simulink model "mdl_4reac"  (R2020b)
settings: Solver=FixedStepAuto  StartTime=0.0  StopTime=stoptime  FixedStep=0.001  MaxStep=1  RelTol=1e-3  AbsTol=1e-6
undefined symbols (not defined in the file or in its folder): p, ref_select, strategy_select
(part 1 of 2)
settings Model: PauseTimes=3  PacingRate=0.100000  Creator=nobel  LastModifiedBy=natha

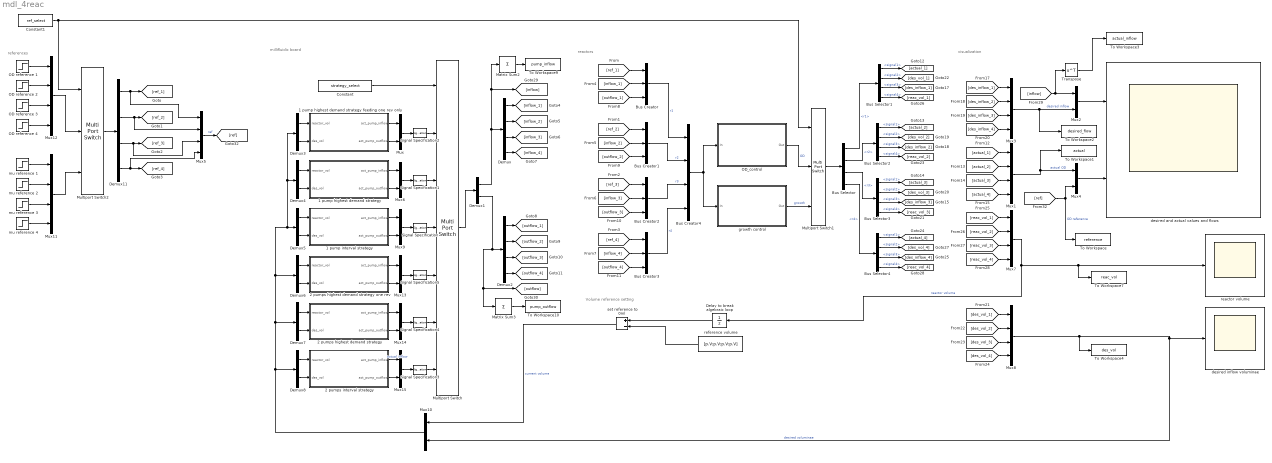
== system mdl_4reac ==
  note: millifluidic board
  note: references
  note: Volume reference setting
  note: visualization
  note: reactors
  " 1 pump highest demand strategy" : Stateflow chart  TreatAsAtomicUnit=on  mask{p=p}
      mask prompts: p "Reactor Parameter Struct"
  " 1 pump highest demand strategy feeding one rev only" : Stateflow chart  TreatAsAtomicUnit=on  mask{p=p}
      mask prompts: p "Reactor Parameter Struct"
  1 pump interval strategy : Stateflow chart  TreatAsAtomicUnit=on  mask{p=p}
      mask prompts: p "Reactor Parameter Struct"
  2 pumps highest demand strategy : Stateflow chart  TreatAsAtomicUnit=on  mask{p=p}
      mask prompts: p "Reactor Parameter Struct"
  2 pumps highest demand strategy one rev : Stateflow chart  TreatAsAtomicUnit=on  mask{p=p}
      mask prompts: p "Reactor Parameter Struct"
  2 pumps interval strategy : Stateflow chart  TreatAsAtomicUnit=on  mask{p=p}
      mask prompts: p "Reactor Parameter Struct"
  Bus Creator{,1..3} (4 alike) : BusCreator  Inputs=3
  Bus Creator4 : BusCreator  Inputs=4
  Bus Selector : BusSelector  OutputSignals=r1,r2,r3,r4
  Bus Selector{1..4} (4 alike) : BusSelector  OutputSignals=signal1,signal2,signal3,signal4
  Constant : Constant  Value=strategy_select
  Constant1 : Constant  Value=ref_select
  Delay to break algebraic loop : UnitDelay  InitialCondition=[15; 15; 15; 15]  SampleTime=-1  HasFrameUpgradeWarning=on
  Demux : Demux
  Demux{1,3..8} (7 alike) : Demux  Outputs=2
  Demux11 : Demux
  Demux2 : Demux
  Matrix Sum2 : Sum  Inputs=+
  Matrix Sum3 : Sum  Inputs=+
  Multiport Switch : MultiPortSwitch  Inputs=6
  Multiport Switch1 : MultiPortSwitch  Inputs=2
  Multiport Switch2 : MultiPortSwitch  Inputs=2
  Mux{,2,4,6,9..10,13..15} (9 alike) : Mux  Inputs=2
  Mux{1,3,5,7..8,11..12} (7 alike) : Mux
  OD reference 1 : Step  Time=p.r1_OD.step_time  Before=p.r1_OD.init_val  After=p.r1_OD.final_val  SampleTime=0  mask{p=p}
      mask prompts: p "Reactor Parameter Struct"
  OD reference 2 : Step  Time=p.r2_OD.step_time  Before=p.r2_OD.init_val  After=p.r2_OD.final_val  SampleTime=0  mask{p=p}
      mask prompts: p "Reactor Parameter Struct"
  OD reference 3 : Step  Time=p.r3_OD.step_time  Before=p.r3_OD.init_val  After=p.r3_OD.final_val  SampleTime=0  mask{p=p}
      mask prompts: p "Reactor Parameter Struct"
  OD reference 4 : Step  Time=p.r4_OD.step_time  Before=p.r4_OD.init_val  After=p.r4_OD.final_val  SampleTime=0  mask{p=p}
      mask prompts: p "Reactor Parameter Struct"
  OD_control : Subsystem
  Signal Specification{,1..5} (6 alike) : SignalSpecification  Dimensions=[8 1]
  To Workspace : ToWorkspace  VariableName=reference  SampleTime=-1
  To Workspace1 : ToWorkspace  VariableName=actual  SampleTime=-1
  To Workspace10 : ToWorkspace  VariableName=pump_outflow  SampleTime=-1
      settings: Save2DSignal=2-D array (concatenate along first dimension)
  To Workspace2 : ToWorkspace  VariableName=desired_flow  SampleTime=-1
  To Workspace3 : ToWorkspace  VariableName=actual_inflow  SampleTime=-1
      settings: Save2DSignal=2-D array (concatenate along first dimension)
  To Workspace4 : ToWorkspace  VariableName=des_vol  SampleTime=-1
  To Workspace7 : ToWorkspace  VariableName=reac_vol  SampleTime=-1
  To Workspace9 : ToWorkspace  VariableName=pump_inflow  SampleTime=-1
      settings: Save2DSignal=2-D array (concatenate along first dimension)
  Transpose : Math  Operator=transpose  SaturateOnIntegerOverflow=on
  desired and actual values and flows : Scope  NumInputPorts=2
  desired inflow voluminae : Scope
  growth control : Subsystem
  mu reference 1 : Step  Time=p.r1_growth.step_time  Before=p.r1_growth.init_val  After=p.r1_growth.final_val  SampleTime=0  mask{p=p}
      mask prompts: p "Reactor Parameter Struct"
  mu reference 2 : Step  Time=p.r2_growth.step_time  Before=p.r2_growth.init_val  After=p.r2_growth.final_val  SampleTime=0  mask{p=p}
      mask prompts: p "Reactor Parameter Struct"
  mu reference 3 : Step  Time=p.r3_growth.step_time  Before=p.r3_growth.init_val  After=p.r3_growth.final_val  SampleTime=0  mask{p=p}
      mask prompts: p "Reactor Parameter Struct"
  mu reference 4 : Step  Time=p.r4_growth.step_time  Before=p.r4_growth.init_val  After=p.r4_growth.final_val  SampleTime=0  mask{p=p}
      mask prompts: p "Reactor Parameter Struct"
  reactor volume : Scope
  reference volume : Constant  Value=[p.V;p.V;p.V;p.V]  mask{p=p}
      mask prompts: p "Reactor Parameter Struct"
  set reference to 0ml : Sum  Inputs=+-
  wires:
  Mux5/1 -> [ref]  "ref"
  Demux11/1 -> Mux5/1, [ref_1]
  Demux11/2 -> Mux5/2, [ref_2]
  Demux11/3 -> Mux5/3, [ref_3]
  Demux11/4 -> Mux5/4, [ref_4]
  Demux/1 -> [inflow_1]
  Demux/2 -> [inflow_2]
  Demux/3 -> [inflow_3]
  Demux/4 -> [inflow_4]
  Demux2/4 -> [outflow_4]
  Demux2/3 -> [outflow_3]
  Demux2/2 -> [outflow_2]
  Demux2/1 -> [outflow_1]
  Demux1/2 -> Matrix Sum3/1, [outflow], Demux2/1
  Matrix Sum2/1 -> To Workspace9/1
  Demux1/1 -> Matrix Sum2/1, [inflow], Demux/1
  Matrix Sum3/1 -> To Workspace10/1
  [des_vol_3] -> Mux8/3
  [ref] -> To Workspace/1, Mux4/2  "OD reference"
  Mux3/1 -> To Workspace2/1, Mux2/2  "desired inflow"
  Delay to break algebraic loop/1 -> set reference to 0ml/1
  Mux8/1 -> To Workspace4/1, Mux10/2, desired inflow voluminae/1  "desired voluminae"
  [des_vol_2] -> Mux8/2
  [reac_vol_1] -> Mux7/1
  [reac_vol_3] -> Mux7/3
  [actual_1] -> Mux1/1
  [actual_4] -> Mux1/4
  Mux4/1 -> desired and actual values and flows/2
  [des_inflow_3] -> Mux3/3
  [des_inflow_2] -> Mux3/2
  reference volume/1 -> set reference to 0ml/2
  Mux1/1 -> To Workspace1/1, Mux4/1  "actual OD"
  [reac_vol_2] -> Mux7/2
  [des_vol_4] -> Mux8/4
  [actual_2] -> Mux1/2
  [inflow] -> Transpose/1, Mux2/1
  [actual_3] -> Mux1/3
  [des_inflow_1] -> Mux3/1
  [reac_vol_4] -> Mux7/4
  set reference to 0ml/1 -> Mux10/1  "current volume"
  [des_vol_1] -> Mux8/1
  Mux2/1 -> desired and actual values and flows/1
  Mux7/1 -> Delay to break algebraic loop/1, To Workspace7/1, reactor volume/1  "reactor volume"
  [des_inflow_4] -> Mux3/4
  Transpose/1 -> To Workspace3/1
  Mux6/1 -> Signal Specification1/1
  Mux/1 -> Signal Specification2/1
  Demux5/1 -> 1 pump interval strategy/1(reactor_vol)
  Demux4/1 -> " 1 pump highest demand strategy"/1(reactor_vol)
  " 1 pump highest demand strategy"/2(act_pump_outflow) -> Mux6/2
  Demux3/2 -> " 1 pump highest demand strategy feeding one rev only"/2(des_vol)
  1 pump interval strategy/1(act_pump_inflow) -> Mux9/1
  " 1 pump highest demand strategy feeding one rev only"/2(act_pump_outflow) -> Mux/2
  " 1 pump highest demand strategy feeding one rev only"/1(act_pump_inflow) -> Mux/1
  1 pump interval strategy/2(act_pump_outflow) -> Mux9/2
  Demux4/2 -> " 1 pump highest demand strategy"/2(des_vol)
  Demux3/1 -> " 1 pump highest demand strategy feeding one rev only"/1(reactor_vol)
  " 1 pump highest demand strategy"/1(act_pump_inflow) -> Mux6/1
  Demux5/2 -> 1 pump interval strategy/2(des_vol)
  Mux9/1 -> Signal Specification/1
  Constant/1 -> Multiport Switch/1
  Bus Selector3/4 -> [reac_vol_3]  "<signal4>"
  Bus Selector4/2 -> [des_vol_4]  "<signal2>"
  Bus Selector3/2 -> [des_vol_3]  "<signal2>"
  Bus Selector1/1 -> [actual_1]  "<signal1>"
  Bus Selector2/3 -> [des_inflow_2]  "<signal3>"
  Bus Selector1/2 -> [des_vol_1]  "<signal2>"
  Bus Selector1/4 -> [reac_vol_1]  "<signal4>"
  Bus Selector1/3 -> [des_inflow_1]  "<signal3>"
  Bus Selector3/3 -> [des_inflow_3]  "<signal3>"
  Bus Selector4/4 -> [reac_vol_4]  "<signal4>"
  Bus Selector2/4 -> [reac_vol_2]  "<signal4>"
  Bus Selector4/3 -> [des_inflow_4]  "<signal3>"
  Bus Selector4/1 -> [actual_4]  "<signal1>"
  Bus Selector3/1 -> [actual_3]  "<signal1>"
  Bus Selector2/1 -> [actual_2]  "<signal1>"
  Bus Selector2/2 -> [des_vol_2]  "<signal2>"
  Bus Selector/2 -> Bus Selector2/1  "<r2>"
  Bus Selector/4 -> Bus Selector4/1  "<r4>"
  [inflow_4] -> Bus Creator3/2
  [inflow_2] -> Bus Creator1/2
  [inflow_1] -> Bus Creator/2
  [inflow_3] -> Bus Creator2/2
  [outflow_3] -> Bus Creator2/3
  [ref_2] -> Bus Creator1/1
  [outflow_1] -> Bus Creator/3
  [ref_1] -> Bus Creator/1
  [outflow_4] -> Bus Creator3/3
  [ref_4] -> Bus Creator3/1
  [ref_3] -> Bus Creator2/1
  [outflow_2] -> Bus Creator1/3
  OD reference 1/1 -> Mux12/1
  OD reference 2/1 -> Mux12/2
  OD reference 3/1 -> Mux12/3
  OD reference 4/1 -> Mux12/4
  mu reference 4/1 -> Mux11/4
  mu reference 3/1 -> Mux11/3
  mu reference 2/1 -> Mux11/2
  mu reference 1/1 -> Mux11/1
  Multiport Switch2/1 -> Demux11/1
  Mux12/1 -> Multiport Switch2/2
  Mux11/1 -> Multiport Switch2/3
  Constant1/1 -> Multiport Switch2/1, Multiport Switch1/1
  Bus Creator/1 -> Bus Creator4/1  "r1"
  Bus Creator1/1 -> Bus Creator4/2  "r2"
  Bus Creator2/1 -> Bus Creator4/3  "r3"
  Bus Creator3/1 -> Bus Creator4/4  "r4"
  Bus Creator4/1 -> growth control/1(In), OD_control/1(In)
  Multiport Switch/1 -> Demux1/1
  Bus Selector/1 -> Bus Selector1/1  "<r1>"
  Bus Selector/3 -> Bus Selector3/1  "<r3>"
  growth control/1(Out) -> Multiport Switch1/3  "growth"
  OD_control/1(Out) -> Multiport Switch1/2  "OD"
  Multiport Switch1/1 -> Bus Selector/1
  Signal Specification/1 -> Multiport Switch/4
  Signal Specification1/1 -> Multiport Switch/3
  Signal Specification2/1 -> Multiport Switch/2
  Demux7/2 -> 2 pumps highest demand strategy/2(des_vol)
  Demux8/1 -> 2 pumps interval strategy/1(reactor_vol)
  Demux6/2 -> 2 pumps highest demand strategy one rev/2(des_vol)
  Mux14/1 -> Signal Specification4/1
  2 pumps highest demand strategy/1(act_pump_inflow) -> Mux14/1
  2 pumps interval strategy/2(act_pump_outflow) -> Mux15/2
  Mux15/1 -> Signal Specification3/1
  Demux7/1 -> 2 pumps highest demand strategy/1(reactor_vol)
  2 pumps highest demand strategy one rev/1(act_pump_inflow) -> Mux13/1
  Mux10/1 -> Demux8/1, Demux7/1, Demux6/1, Demux5/1, Demux4/1, Demux3/1
  2 pumps highest demand strategy/2(act_pump_outflow) -> Mux14/2
  Demux6/1 -> 2 pumps highest demand strategy one rev/1(reactor_vol)
  Demux8/2 -> 2 pumps interval strategy/2(des_vol)
  2 pumps highest demand strategy one rev/2(act_pump_outflow) -> Mux13/2
  2 pumps interval strategy/1(act_pump_inflow) -> Mux15/1  "actual inflow"
  Mux13/1 -> Signal Specification5/1
  Signal Specification3/1 -> Multiport Switch/7
  Signal Specification5/1 -> Multiport Switch/5
  Signal Specification4/1 -> Multiport Switch/6

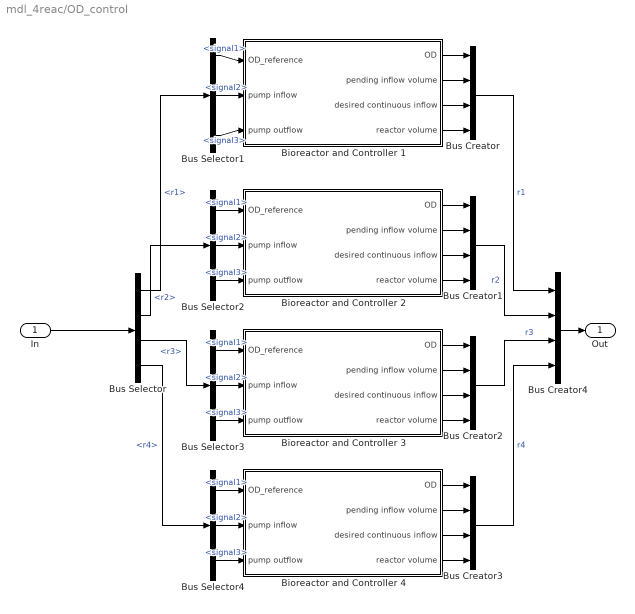
== system mdl_4reac/OD_control ==
  In : Inport
  Bioreactor and Controller 1 : Subsystem  mask{p=p}
      mask prompts: p "Reactor Parameter Struct"
  Bioreactor and Controller 2 : Subsystem  mask{p=p}
      mask prompts: p "Reactor Parameter Struct"
  Bioreactor and Controller 3 : Subsystem  mask{p=p}
      mask prompts: p "Reactor Parameter Struct"
  Bioreactor and Controller 4 : Subsystem  mask{p=p}
      mask prompts: p "Reactor Parameter Struct"
  Bus Creator{,1..4} (5 alike) : BusCreator  Inputs=4
  Bus Selector : BusSelector  OutputSignals=r1,r2,r3,r4
  Bus Selector{1..4} (4 alike) : BusSelector  OutputSignals=signal1,signal2,signal3
  Out : Outport
  wires:
  Bus Selector4/1 -> Bioreactor and Controller 4/1(OD_reference)  "<signal1>"
  Bus Selector/1 -> Bus Selector1/1  "<r1>"
  Bus Selector2/2 -> Bioreactor and Controller 2/2(pump inflow)  "<signal2>"
  Bus Creator3/1 -> Bus Creator4/4  "r4"
  Bioreactor and Controller 4/2(pending inflow volume) -> Bus Creator3/2
  Bus Selector1/2 -> Bioreactor and Controller 1/2(pump inflow)  "<signal2>"
  Bus Selector3/2 -> Bioreactor and Controller 3/2(pump inflow)  "<signal2>"
  Bus Selector/2 -> Bus Selector2/1  "<r2>"
  Bus Selector1/3 -> Bioreactor and Controller 1/3(pump outflow)  "<signal3>"
  Bus Creator4/1 -> Out/1
  Bus Selector/4 -> Bus Selector4/1  "<r4>"
  Bioreactor and Controller 2/4(reactor volume) -> Bus Creator1/4
  Bioreactor and Controller 2/1(OD) -> Bus Creator1/1
  Bioreactor and Controller 4/4(reactor volume) -> Bus Creator3/4
  Bus Selector2/3 -> Bioreactor and Controller 2/3(pump outflow)  "<signal3>"
  Bus Selector3/3 -> Bioreactor and Controller 3/3(pump outflow)  "<signal3>"
  Bioreactor and Controller 3/3(desired continuous inflow) -> Bus Creator2/3
  Bioreactor and Controller 1/1(OD) -> Bus Creator/1
  Bus Selector1/1 -> Bioreactor and Controller 1/1(OD_reference)  "<signal1>"
  Bioreactor and Controller 4/3(desired continuous inflow) -> Bus Creator3/3
  Bioreactor and Controller 2/3(desired continuous inflow) -> Bus Creator1/3
  Bus Selector3/1 -> Bioreactor and Controller 3/1(OD_reference)  "<signal1>"
  Bioreactor and Controller 3/4(reactor volume) -> Bus Creator2/4
  Bioreactor and Controller 4/1(OD) -> Bus Creator3/1
  Bioreactor and Controller 1/4(reactor volume) -> Bus Creator/4
  Bioreactor and Controller 3/2(pending inflow volume) -> Bus Creator2/2
  Bioreactor and Controller 3/1(OD) -> Bus Creator2/1
  Bioreactor and Controller 1/2(pending inflow volume) -> Bus Creator/2
  Bus Creator2/1 -> Bus Creator4/3  "r3"
  Bus Creator/1 -> Bus Creator4/1  "r1"
  Bus Selector4/3 -> Bioreactor and Controller 4/3(pump outflow)  "<signal3>"
  Bus Selector4/2 -> Bioreactor and Controller 4/2(pump inflow)  "<signal2>"
  Bus Selector/3 -> Bus Selector3/1  "<r3>"
  Bioreactor and Controller 1/3(desired continuous inflow) -> Bus Creator/3
  Bioreactor and Controller 2/2(pending inflow volume) -> Bus Creator1/2
  Bus Creator1/1 -> Bus Creator4/2  "r2"
  In/1 -> Bus Selector/1
  Bus Selector2/1 -> Bioreactor and Controller 2/1(OD_reference)  "<signal1>"

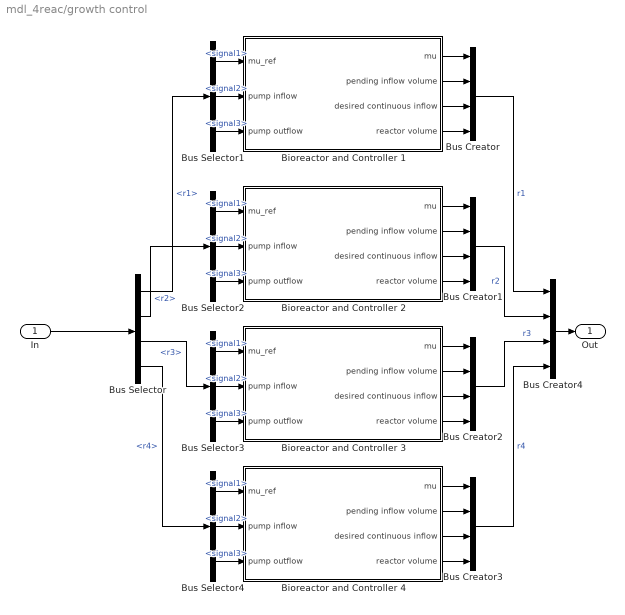
== system mdl_4reac/growth control ==
  In : Inport
  Bioreactor and Controller 1 : Subsystem  mask{p=p}
      mask prompts: p "Reactor Parameter Struct"
  Bioreactor and Controller 2 : Subsystem  mask{p=p}
      mask prompts: p "Reactor Parameter Struct"
  Bioreactor and Controller 3 : Subsystem  mask{p=p}
      mask prompts: p "Reactor Parameter Struct"
  Bioreactor and Controller 4 : Subsystem  mask{p=p}
      mask prompts: p "Reactor Parameter Struct"
  Bus Creator{,1..4} (5 alike) : BusCreator  Inputs=4
  Bus Selector : BusSelector  OutputSignals=r1,r2,r3,r4
  Bus Selector{1..4} (4 alike) : BusSelector  OutputSignals=signal1,signal2,signal3
  Out : Outport
  wires:
  Bus Creator2/1 -> Bus Creator4/3  "r3"
  Bus Creator/1 -> Bus Creator4/1  "r1"
  Bus Creator1/1 -> Bus Creator4/2  "r2"
  Bus Selector/3 -> Bus Selector3/1  "<r3>"
  In/1 -> Bus Selector/1
  Bus Selector2/3 -> Bioreactor and Controller 2/3(pump outflow)  "<signal3>"
  Bioreactor and Controller 3/2(pending inflow volume) -> Bus Creator2/2
  Bus Selector3/3 -> Bioreactor and Controller 3/3(pump outflow)  "<signal3>"
  Bioreactor and Controller 3/4(reactor volume) -> Bus Creator2/4
  Bioreactor and Controller 3/3(desired continuous inflow) -> Bus Creator2/3
  Bus Selector3/1 -> Bioreactor and Controller 3/1(mu_ref)  "<signal1>"
  Bus Selector3/2 -> Bioreactor and Controller 3/2(pump inflow)  "<signal2>"
  Bioreactor and Controller 2/2(pending inflow volume) -> Bus Creator1/2
  Bus Selector2/2 -> Bioreactor and Controller 2/2(pump inflow)  "<signal2>"
  Bus Selector2/1 -> Bioreactor and Controller 2/1(mu_ref)  "<signal1>"
  Bioreactor and Controller 2/3(desired continuous inflow) -> Bus Creator1/3
  Bioreactor and Controller 2/4(reactor volume) -> Bus Creator1/4
  Bioreactor and Controller 2/1(mu) -> Bus Creator1/1
  Bus Selector/4 -> Bus Selector4/1  "<r4>"
  Bioreactor and Controller 4/4(reactor volume) -> Bus Creator3/4
  Bioreactor and Controller 4/3(desired continuous inflow) -> Bus Creator3/3
  Bioreactor and Controller 4/2(pending inflow volume) -> Bus Creator3/2
  Bus Selector1/1 -> Bioreactor and Controller 1/1(mu_ref)  "<signal1>"
  Bus Selector4/1 -> Bioreactor and Controller 4/1(mu_ref)  "<signal1>"
  Bus Selector4/3 -> Bioreactor and Controller 4/3(pump outflow)  "<signal3>"
  Bus Selector4/2 -> Bioreactor and Controller 4/2(pump inflow)  "<signal2>"
  Bioreactor and Controller 4/1(mu) -> Bus Creator3/1
  Bioreactor and Controller 1/4(reactor volume) -> Bus Creator/4
  Bioreactor and Controller 1/3(desired continuous inflow) -> Bus Creator/3
  Bioreactor and Controller 1/1(mu) -> Bus Creator/1
  Bus Selector1/2 -> Bioreactor and Controller 1/2(pump inflow)  "<signal2>"
  Bus Selector/1 -> Bus Selector1/1  "<r1>"
  Bus Creator3/1 -> Bus Creator4/4  "r4"
  Bus Selector/2 -> Bus Selector2/1  "<r2>"
  Bus Selector1/3 -> Bioreactor and Controller 1/3(pump outflow)  "<signal3>"
  Bioreactor and Controller 1/2(pending inflow volume) -> Bus Creator/2
  Bioreactor and Controller 3/1(mu) -> Bus Creator2/1
  Bus Creator4/1 -> Out/1

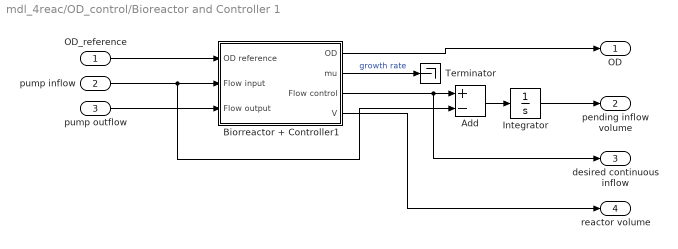
== system mdl_4reac/OD_control/Bioreactor and Controller 1 ==
  OD_reference : Inport
  pump inflow : Inport  Port=2
  pump outflow : Inport  Port=3
  Add : Sum  Inputs=+-
  Biorreactor + Controller1 : Subsystem
  Integrator : Integrator
  Terminator : Terminator
  OD : Outport
  pending inflow volume : Outport  Port=2
  desired continuous inflow : Outport  Port=3
  reactor volume : Outport  Port=4
  wires:
  OD_reference/1 -> Biorreactor + Controller1/1(OD reference)
  Biorreactor + Controller1/2(mu) -> Terminator/1  "growth rate"
  Biorreactor + Controller1/1(OD) -> OD/1
  Biorreactor + Controller1/3(Flow control) -> desired continuous inflow/1, Add/1
  pump inflow/1 -> Add/2, Biorreactor + Controller1/2(Flow input)
  Biorreactor + Controller1/4(V) -> reactor volume/1
  pump outflow/1 -> Biorreactor + Controller1/3(Flow output)
  Add/1 -> Integrator/1
  Integrator/1 -> pending inflow volume/1

== system mdl_4reac/OD_control/Bioreactor and Controller 2 ==
  OD_reference : Inport
  pump inflow : Inport  Port=2
  pump outflow : Inport  Port=3
  Add : Sum  Inputs=+-
  Biorreactor + Controller1 : Subsystem
  Integrator : Integrator
  Terminator : Terminator
  OD : Outport
  pending inflow volume : Outport  Port=2
  desired continuous inflow : Outport  Port=3
  reactor volume : Outport  Port=4
  wires:
  Integrator/1 -> pending inflow volume/1
  Add/1 -> Integrator/1
  pump outflow/1 -> Biorreactor + Controller1/3(Flow output)
  Biorreactor + Controller1/4(V) -> reactor volume/1
  pump inflow/1 -> Biorreactor + Controller1/2(Flow input), Add/2
  Biorreactor + Controller1/3(Flow control) -> Add/1, desired continuous inflow/1
  Biorreactor + Controller1/1(OD) -> OD/1
  Biorreactor + Controller1/2(mu) -> Terminator/1  "growth rate"
  OD_reference/1 -> Biorreactor + Controller1/1(OD reference)

== system mdl_4reac/OD_control/Bioreactor and Controller 3 ==
  OD_reference : Inport
  pump inflow : Inport  Port=2
  pump outflow : Inport  Port=3
  Add : Sum  Inputs=+-
  Biorreactor + Controller1 : Subsystem
  Integrator : Integrator
  Terminator : Terminator
  OD : Outport
  pending inflow volume : Outport  Port=2
  desired continuous inflow : Outport  Port=3
  reactor volume : Outport  Port=4
  wires:
  OD_reference/1 -> Biorreactor + Controller1/1(OD reference)
  Biorreactor + Controller1/2(mu) -> Terminator/1  "growth rate"
  Biorreactor + Controller1/1(OD) -> OD/1
  Biorreactor + Controller1/3(Flow control) -> desired continuous inflow/1, Add/1
  pump inflow/1 -> Add/2, Biorreactor + Controller1/2(Flow input)
  Biorreactor + Controller1/4(V) -> reactor volume/1
  pump outflow/1 -> Biorreactor + Controller1/3(Flow output)
  Add/1 -> Integrator/1
  Integrator/1 -> pending inflow volume/1

== system mdl_4reac/OD_control/Bioreactor and Controller 4 ==
  OD_reference : Inport
  pump inflow : Inport  Port=2
  pump outflow : Inport  Port=3
  Add : Sum  Inputs=+-
  Biorreactor + Controller1 : Subsystem
  Integrator : Integrator
  Terminator : Terminator
  OD : Outport
  pending inflow volume : Outport  Port=2
  desired continuous inflow : Outport  Port=3
  reactor volume : Outport  Port=4
  wires:
  Integrator/1 -> pending inflow volume/1
  Add/1 -> Integrator/1
  pump outflow/1 -> Biorreactor + Controller1/3(Flow output)
  Biorreactor + Controller1/4(V) -> reactor volume/1
  pump inflow/1 -> Biorreactor + Controller1/2(Flow input), Add/2
  Biorreactor + Controller1/3(Flow control) -> Add/1, desired continuous inflow/1
  Biorreactor + Controller1/1(OD) -> OD/1
  Biorreactor + Controller1/2(mu) -> Terminator/1  "growth rate"
  OD_reference/1 -> Biorreactor + Controller1/1(OD reference)

== system mdl_4reac/growth control/Bioreactor and Controller 1 ==
  mu_ref : Inport
  pump inflow : Inport  Port=2
  pump outflow : Inport  Port=3
  Add : Sum  Inputs=+-
  Biorreactor + Controller 1 : Subsystem
  Integrator : Integrator
  Terminator1 : Terminator
  mu : Outport
  pending inflow volume : Outport  Port=2
  desired continuous inflow : Outport  Port=3
  reactor volume : Outport  Port=4
  wires:
  pump inflow/1 -> Add/2, Biorreactor + Controller 1/2(Flow input)
  mu_ref/1 -> Biorreactor + Controller 1/1(mu reference)
  pump outflow/1 -> Biorreactor + Controller 1/3(Flow output)
  Biorreactor + Controller 1/1(OD) -> Terminator1/1
  Biorreactor + Controller 1/2(mu) -> mu/1
  Add/1 -> Integrator/1
  Integrator/1 -> pending inflow volume/1
  Biorreactor + Controller 1/3(Flow control) -> Add/1, desired continuous inflow/1
  Biorreactor + Controller 1/4(V) -> reactor volume/1

== system mdl_4reac/growth control/Bioreactor and Controller 2 ==
  mu_ref : Inport
  pump inflow : Inport  Port=2
  pump outflow : Inport  Port=3
  Add : Sum  Inputs=+-
  Biorreactor + Controller 1 : Subsystem
  Integrator : Integrator
  Terminator1 : Terminator
  mu : Outport
  pending inflow volume : Outport  Port=2
  desired continuous inflow : Outport  Port=3
  reactor volume : Outport  Port=4
  wires:
  Biorreactor + Controller 1/4(V) -> reactor volume/1
  Biorreactor + Controller 1/3(Flow control) -> desired continuous inflow/1, Add/1
  Integrator/1 -> pending inflow volume/1
  Add/1 -> Integrator/1
  Biorreactor + Controller 1/2(mu) -> mu/1
  Biorreactor + Controller 1/1(OD) -> Terminator1/1
  pump outflow/1 -> Biorreactor + Controller 1/3(Flow output)
  mu_ref/1 -> Biorreactor + Controller 1/1(mu reference)
  pump inflow/1 -> Biorreactor + Controller 1/2(Flow input), Add/2

== system mdl_4reac/growth control/Bioreactor and Controller 3 ==
  mu_ref : Inport
  pump inflow : Inport  Port=2
  pump outflow : Inport  Port=3
  Add : Sum  Inputs=+-
  Biorreactor + Controller 1 : Subsystem
  Integrator : Integrator
  Terminator1 : Terminator
  mu : Outport
  pending inflow volume : Outport  Port=2
  desired continuous inflow : Outport  Port=3
  reactor volume : Outport  Port=4
  wires:
  pump inflow/1 -> Add/2, Biorreactor + Controller 1/2(Flow input)
  mu_ref/1 -> Biorreactor + Controller 1/1(mu reference)
  pump outflow/1 -> Biorreactor + Controller 1/3(Flow output)
  Biorreactor + Controller 1/1(OD) -> Terminator1/1
  Biorreactor + Controller 1/2(mu) -> mu/1
  Add/1 -> Integrator/1
  Integrator/1 -> pending inflow volume/1
  Biorreactor + Controller 1/3(Flow control) -> Add/1, desired continuous inflow/1
  Biorreactor + Controller 1/4(V) -> reactor volume/1

== system mdl_4reac/growth control/Bioreactor and Controller 4 ==
  mu_ref : Inport
  pump inflow : Inport  Port=2
  pump outflow : Inport  Port=3
  Add : Sum  Inputs=+-
  Biorreactor + Controller 1 : Subsystem
  Integrator : Integrator
  Terminator1 : Terminator
  mu : Outport
  pending inflow volume : Outport  Port=2
  desired continuous inflow : Outport  Port=3
  reactor volume : Outport  Port=4
  wires:
  Biorreactor + Controller 1/4(V) -> reactor volume/1
  Biorreactor + Controller 1/3(Flow control) -> desired continuous inflow/1, Add/1
  Integrator/1 -> pending inflow volume/1
  Add/1 -> Integrator/1
  Biorreactor + Controller 1/2(mu) -> mu/1
  Biorreactor + Controller 1/1(OD) -> Terminator1/1
  pump outflow/1 -> Biorreactor + Controller 1/3(Flow output)
  mu_ref/1 -> Biorreactor + Controller 1/1(mu reference)
  pump inflow/1 -> Biorreactor + Controller 1/2(Flow input), Add/2

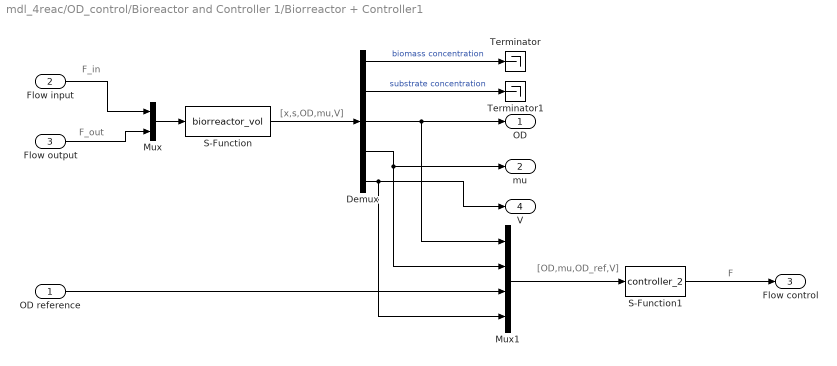
== system mdl_4reac/OD_control/Bioreactor and Controller 1/Biorreactor + Controller1 ==
  note: F_out
  note: [OD,mu,OD_ref,V]
  note: F
  note: [x,s,OD,mu,V]
  note: F_in
  OD reference : Inport
  Flow input : Inport  Port=2
  Flow output : Inport  Port=3
  Demux : Demux  Outputs=5
  Mux : Mux  Inputs=2
  Mux1 : Mux
  S-Function : S-Function  FunctionName=biorreactor_vol  Parameters=[0.1 16 15],p  SFunctionDeploymentMode=off  EnableBusSupport=off
  S-Function1 : S-Function  FunctionName=controller_2  Parameters=p  SFunctionDeploymentMode=off  EnableBusSupport=off
  Terminator : Terminator
  Terminator1 : Terminator
  OD : Outport
  mu : Outport  Port=2
  Flow control : Outport  Port=3
  V : Outport  Port=4
  wires:
  Demux/4 -> Mux1/2, mu/1
  Demux/3 -> Mux1/1, OD/1
  OD reference/1 -> Mux1/3
  S-Function/1 -> Demux/1
  Demux/2 -> Terminator1/1  "substrate concentration"
  Mux1/1 -> S-Function1/1
  S-Function1/1 -> Flow control/1
  Demux/1 -> Terminator/1  "biomass concentration"
  Demux/5 -> Mux1/4, V/1
  Mux/1 -> S-Function/1
  Flow input/1 -> Mux/1
  Flow output/1 -> Mux/2

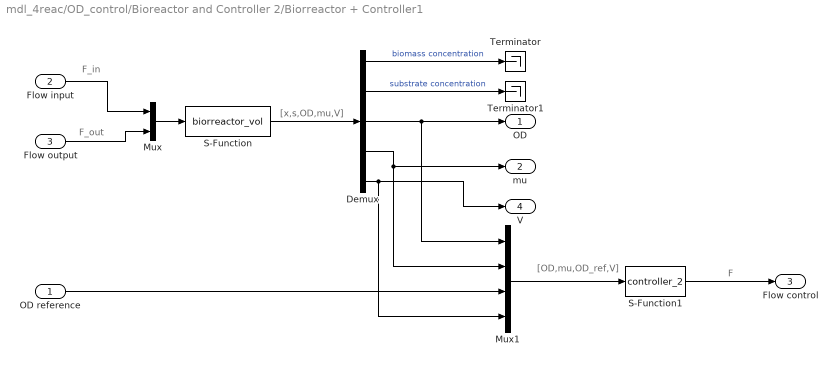
== system mdl_4reac/OD_control/Bioreactor and Controller 2/Biorreactor + Controller1 ==
  note: F_in
  note: [x,s,OD,mu,V]
  note: F
  note: [OD,mu,OD_ref,V]
  note: F_out
  OD reference : Inport
  Flow input : Inport  Port=2
  Flow output : Inport  Port=3
  Demux : Demux  Outputs=5
  Mux : Mux  Inputs=2
  Mux1 : Mux
  S-Function : S-Function  FunctionName=biorreactor_vol  Parameters=[0.1 16 15],p  SFunctionDeploymentMode=off  EnableBusSupport=off
  S-Function1 : S-Function  FunctionName=controller_2  Parameters=p  SFunctionDeploymentMode=off  EnableBusSupport=off
  Terminator : Terminator
  Terminator1 : Terminator
  OD : Outport
  mu : Outport  Port=2
  Flow control : Outport  Port=3
  V : Outport  Port=4
  wires:
  Flow output/1 -> Mux/2
  Flow input/1 -> Mux/1
  Mux/1 -> S-Function/1
  Demux/5 -> V/1, Mux1/4
  Demux/1 -> Terminator/1  "biomass concentration"
  S-Function1/1 -> Flow control/1
  Mux1/1 -> S-Function1/1
  Demux/2 -> Terminator1/1  "substrate concentration"
  S-Function/1 -> Demux/1
  OD reference/1 -> Mux1/3
  Demux/3 -> OD/1, Mux1/1
  Demux/4 -> mu/1, Mux1/2

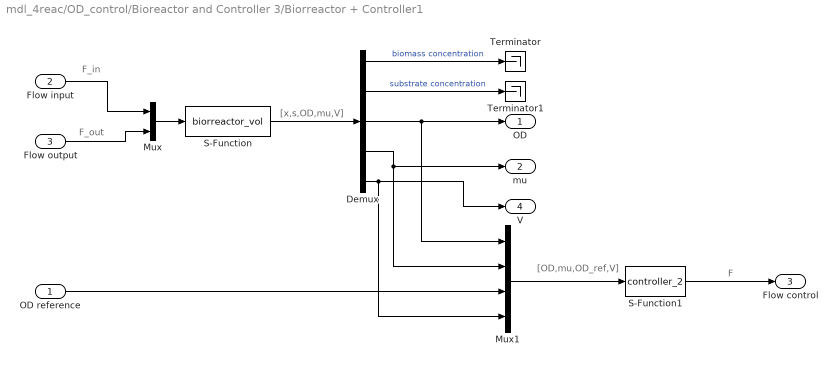
== system mdl_4reac/OD_control/Bioreactor and Controller 3/Biorreactor + Controller1 ==
  note: F_out
  note: [OD,mu,OD_ref,V]
  note: F
  note: [x,s,OD,mu,V]
  note: F_in
  OD reference : Inport
  Flow input : Inport  Port=2
  Flow output : Inport  Port=3
  Demux : Demux  Outputs=5
  Mux : Mux  Inputs=2
  Mux1 : Mux
  S-Function : S-Function  FunctionName=biorreactor_vol  Parameters=[0.1 16 15],p  SFunctionDeploymentMode=off  EnableBusSupport=off
  S-Function1 : S-Function  FunctionName=controller_2  Parameters=p  SFunctionDeploymentMode=off  EnableBusSupport=off
  Terminator : Terminator
  Terminator1 : Terminator
  OD : Outport
  mu : Outport  Port=2
  Flow control : Outport  Port=3
  V : Outport  Port=4
  wires:
  Demux/4 -> Mux1/2, mu/1
  Demux/3 -> Mux1/1, OD/1
  OD reference/1 -> Mux1/3
  S-Function/1 -> Demux/1
  Demux/2 -> Terminator1/1  "substrate concentration"
  Mux1/1 -> S-Function1/1
  S-Function1/1 -> Flow control/1
  Demux/1 -> Terminator/1  "biomass concentration"
  Demux/5 -> Mux1/4, V/1
  Mux/1 -> S-Function/1
  Flow input/1 -> Mux/1
  Flow output/1 -> Mux/2

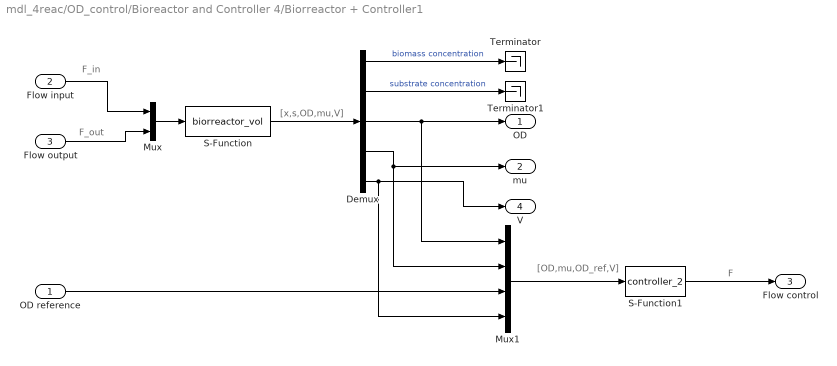
== system mdl_4reac/OD_control/Bioreactor and Controller 4/Biorreactor + Controller1 ==
  note: F_in
  note: [x,s,OD,mu,V]
  note: F
  note: [OD,mu,OD_ref,V]
  note: F_out
  OD reference : Inport
  Flow input : Inport  Port=2
  Flow output : Inport  Port=3
  Demux : Demux  Outputs=5
  Mux : Mux  Inputs=2
  Mux1 : Mux
  S-Function : S-Function  FunctionName=biorreactor_vol  Parameters=[0.1 16 15],p  SFunctionDeploymentMode=off  EnableBusSupport=off
  S-Function1 : S-Function  FunctionName=controller_2  Parameters=p  SFunctionDeploymentMode=off  EnableBusSupport=off
  Terminator : Terminator
  Terminator1 : Terminator
  OD : Outport
  mu : Outport  Port=2
  Flow control : Outport  Port=3
  V : Outport  Port=4
  wires:
  Flow output/1 -> Mux/2
  Flow input/1 -> Mux/1
  Mux/1 -> S-Function/1
  Demux/5 -> V/1, Mux1/4
  Demux/1 -> Terminator/1  "biomass concentration"
  S-Function1/1 -> Flow control/1
  Mux1/1 -> S-Function1/1
  Demux/2 -> Terminator1/1  "substrate concentration"
  S-Function/1 -> Demux/1
  OD reference/1 -> Mux1/3
  Demux/3 -> OD/1, Mux1/1
  Demux/4 -> mu/1, Mux1/2

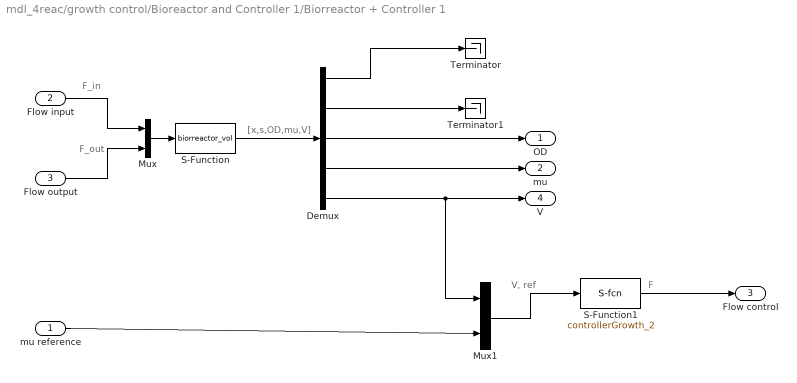
== system mdl_4reac/growth control/Bioreactor and Controller 1/Biorreactor + Controller 1 ==
  note: F_out
  note: V, ref
  note: F
  note: [x,s,OD,mu,V]
  note: F_in
  mu reference : Inport
  Flow input : Inport  Port=2
  Flow output : Inport  Port=3
  Demux : Demux  Outputs=5
  Mux : Mux  Inputs=2
  Mux1 : Mux  Inputs=2
  S-Function : S-Function  FunctionName=biorreactor_vol  Parameters=[0.1 16 15],p  SFunctionDeploymentMode=off  EnableBusSupport=off
  S-Function1 : S-Function  FunctionName=controllerGrowth_2  Parameters=p  SFunctionDeploymentMode=off  EnableBusSupport=off
  Terminator : Terminator
  Terminator1 : Terminator
  OD : Outport
  mu : Outport  Port=2
  Flow control : Outport  Port=3
  V : Outport  Port=4
  wires:
  Demux/4 -> mu/1
  Demux/3 -> OD/1
  mu reference/1 -> Mux1/2
  S-Function/1 -> Demux/1
  Demux/2 -> Terminator1/1
  Mux1/1 -> S-Function1/1
  S-Function1/1 -> Flow control/1
  Demux/1 -> Terminator/1
  Mux/1 -> S-Function/1
  Flow input/1 -> Mux/1
  Flow output/1 -> Mux/2
  Demux/5 -> Mux1/1, V/1

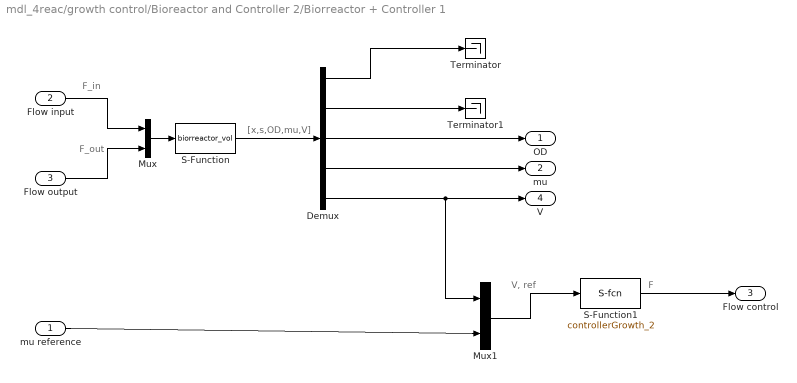
== system mdl_4reac/growth control/Bioreactor and Controller 2/Biorreactor + Controller 1 ==
  note: F_in
  note: [x,s,OD,mu,V]
  note: F
  note: V, ref
  note: F_out
  mu reference : Inport
  Flow input : Inport  Port=2
  Flow output : Inport  Port=3
  Demux : Demux  Outputs=5
  Mux : Mux  Inputs=2
  Mux1 : Mux  Inputs=2
  S-Function : S-Function  FunctionName=biorreactor_vol  Parameters=[0.1 16 15],p  SFunctionDeploymentMode=off  EnableBusSupport=off
  S-Function1 : S-Function  FunctionName=controllerGrowth_2  Parameters=p  SFunctionDeploymentMode=off  EnableBusSupport=off
  Terminator : Terminator
  Terminator1 : Terminator
  OD : Outport
  mu : Outport  Port=2
  Flow control : Outport  Port=3
  V : Outport  Port=4
  wires:
  Demux/5 -> V/1, Mux1/1
  Flow output/1 -> Mux/2
  Flow input/1 -> Mux/1
  Mux/1 -> S-Function/1
  Demux/1 -> Terminator/1
  S-Function1/1 -> Flow control/1
  Mux1/1 -> S-Function1/1
  Demux/2 -> Terminator1/1
  S-Function/1 -> Demux/1
  mu reference/1 -> Mux1/2
  Demux/3 -> OD/1
  Demux/4 -> mu/1

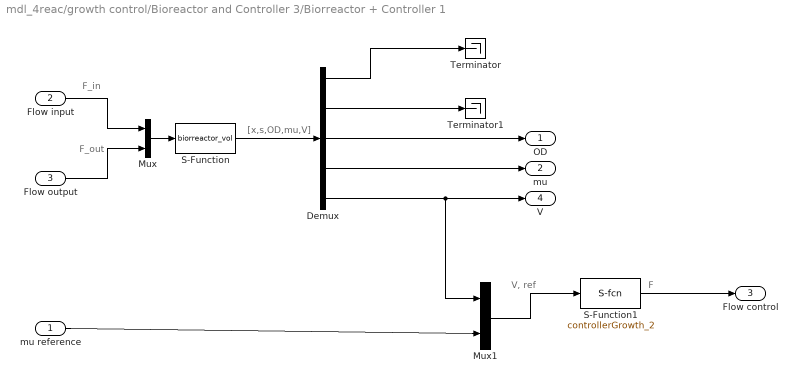
== system mdl_4reac/growth control/Bioreactor and Controller 3/Biorreactor + Controller 1 ==
  note: F_out
  note: V, ref
  note: F
  note: [x,s,OD,mu,V]
  note: F_in
  mu reference : Inport
  Flow input : Inport  Port=2
  Flow output : Inport  Port=3
  Demux : Demux  Outputs=5
  Mux : Mux  Inputs=2
  Mux1 : Mux  Inputs=2
  S-Function : S-Function  FunctionName=biorreactor_vol  Parameters=[0.1 16 15],p  SFunctionDeploymentMode=off  EnableBusSupport=off
  S-Function1 : S-Function  FunctionName=controllerGrowth_2  Parameters=p  SFunctionDeploymentMode=off  EnableBusSupport=off
  Terminator : Terminator
  Terminator1 : Terminator
  OD : Outport
  mu : Outport  Port=2
  Flow control : Outport  Port=3
  V : Outport  Port=4
  wires:
  Demux/4 -> mu/1
  Demux/3 -> OD/1
  mu reference/1 -> Mux1/2
  S-Function/1 -> Demux/1
  Demux/2 -> Terminator1/1
  Mux1/1 -> S-Function1/1
  S-Function1/1 -> Flow control/1
  Demux/1 -> Terminator/1
  Mux/1 -> S-Function/1
  Flow input/1 -> Mux/1
  Flow output/1 -> Mux/2
  Demux/5 -> Mux1/1, V/1

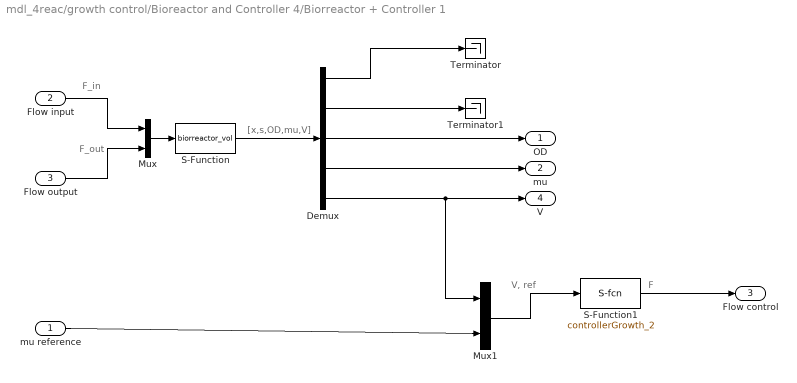
== system mdl_4reac/growth control/Bioreactor and Controller 4/Biorreactor + Controller 1 ==
  note: F_in
  note: [x,s,OD,mu,V]
  note: F
  note: V, ref
  note: F_out
  mu reference : Inport
  Flow input : Inport  Port=2
  Flow output : Inport  Port=3
  Demux : Demux  Outputs=5
  Mux : Mux  Inputs=2
  Mux1 : Mux  Inputs=2
  S-Function : S-Function  FunctionName=biorreactor_vol  Parameters=[0.1 16 15],p  SFunctionDeploymentMode=off  EnableBusSupport=off
  S-Function1 : S-Function  FunctionName=controllerGrowth_2  Parameters=p  SFunctionDeploymentMode=off  EnableBusSupport=off
  Terminator : Terminator
  Terminator1 : Terminator
  OD : Outport
  mu : Outport  Port=2
  Flow control : Outport  Port=3
  V : Outport  Port=4
  wires:
  Demux/5 -> V/1, Mux1/1
  Flow output/1 -> Mux/2
  Flow input/1 -> Mux/1
  Mux/1 -> S-Function/1
  Demux/1 -> Terminator/1
  S-Function1/1 -> Flow control/1
  Mux1/1 -> S-Function1/1
  Demux/2 -> Terminator1/1
  S-Function/1 -> Demux/1
  mu reference/1 -> Mux1/2
  Demux/3 -> OD/1
  Demux/4 -> mu/1

== stateflow chart mdl_4reac/1 pump interval strategy ==
  state procedures [parallel]
    settings: executionOrder=3
    state normal
    state sampling
      entry: sampling_req=true;
    (default) -> normal
    normal -> sampling : after(15, sec)
    sampling -> normal : sampling_done
  state counter [parallel]
    settings: executionOrder=1
    state init_counter
      entry: reac_ind = 1;
    state increase_counter
      entry: reac_ind = reac_ind+1;
    state cycle_over
    (default) -> init_counter : % loop_counter
    increase_counter -> (junction 211) : after(p.interval/p.num_reac,sec)
    (junction 211) -> cycle_over [order 2]
    (junction 211) -> increase_counter [order 1] : [reac_ind<p.num_reac]
    init_counter -> increase_counter : after(p.interval/p.num_reac,sec)
    cycle_over -> init_counter : next_cycle
  state feeding_wasting_sampling [parallel]
    settings: executionOrder=2
    state inflow
      state inflow_act
        entry: vol_pump_in=floor(des_vol(reac_ind)/...
        p.pump_res)*p.pump_res;
        act_pump_inflow(reac_ind)=p.max_pump_flow;
      state inflow_inact
        entry: act_pump_inflow=zeros(4,1);
      inflow_act -> inflow_inact [order 3] : [vol_pump_in<=0]
      inflow_act -> inflow_inact [order 1] : after(vol_pump_in/p.max_pump_flow,sec)
      inflow_inact -> inflow_act [order 1] : enter(counter.increase_counter)
      inflow_act -> inflow_inact [order 2] : after(p.interval/p.num_reac-1e-3,sec)
    state outflow_waste
      state outflow_act
        entry: vol_pump_out=reactor_vol(reac_ind);
        act_pump_outflow(reac_ind)=p.max_pump_flow;
      state outflow_inact
        entry: act_pump_outflow=zeros(4,1);
      feeding_wasting_sampling.outflow_waste.outflow_act -> feeding_wasting_sampling.outflow_waste.outflow_inact [order 3] : [vol_pump_out<=0]
      feeding_wasting_sampling.outflow_waste.outflow_act -> feeding_wasting_sampling.outflow_waste.outflow_inact [order 1] : after(vol_pump_out/p.max_pump_flow,sec)
      feeding_wasting_sampling.outflow_waste.outflow_inact -> feeding_wasting_sampling.outflow_waste.outflow_act [order 1] : enter(counter.increase_counter)
      feeding_wasting_sampling.outflow_waste.outflow_act -> feeding_wasting_sampling.outflow_waste.outflow_inact [order 2] : after(p.interval/p.num_reac-1e-3,sec)
    state cleaning_procedure
    state outflow_sampling
      state outflow_act
        entry: vol_pump_out=p.pump_res;
        act_pump_outflow(reac_ind)=p.max_pump_flow;
      state outflow_inact
        entry: act_pump_outflow=zeros(4,1);
      feeding_wasting_sampling.outflow_sampling.outflow_act -> feeding_wasting_sampling.outflow_sampling.outflow_inact : after(vol_pump_out/p.max_pump_flow,sec)
      feeding_wasting_sampling.outflow_sampling.outflow_inact -> feeding_wasting_sampling.outflow_sampling.outflow_act [order 1] : enter(counter.increase_counter)
    (default) -> inflow_act
    (junction 263) -> inflow_act [order 2] : [in(procedures.normal)]{send(next_cycle,counter)}
    inflow_inact -> feeding_wasting_sampling.outflow_waste.outflow_act [order 2] : enter(counter.cycle_over) {send(next_cycle,counter)}
    feeding_wasting_sampling.outflow_waste.outflow_inact -> inflow_act [order 3] : [enter(counter.cycle_over) && in(procedures.normal)]{send(next_cycle,counter)}
    feeding_wasting_sampling.outflow_waste.outflow_inact -> cleaning_procedure [order 2] : [enter(counter.cycle_over)]
    feeding_wasting_sampling.outflow_sampling.outflow_inact -> cleaning_procedure [order 2] : [enter(counter.cycle_over)]{send(sampling_done, procedures)}
    cleaning_procedure -> (junction 263) : after(p.clean_time,sec)
    (junction 263) -> feeding_wasting_sampling.outflow_sampling.outflow_act [order 1] : [in(procedures.sampling)] {send(next_cycle,counter)}
  data: act_pump_inflow output =[0;0;0;0]; reactor_vol input; des_vol input size=4; vol_pump_in local; act_pump_outflow output =[0;0;0;0]; vol_pump_out local; reac_ind local; sampling_req local; p parameter
  events: sampling_done local FUNCTION_CALL_EVENT; next_cycle local FUNCTION_CALL_EVENT

== stateflow chart mdl_4reac/ 1 pump highest demand strategy ==
  state procedures [parallel]
    settings: executionOrder=2
    state normal
    state sampling
      entry: sampling_req=true;
    (default) -> normal
    normal -> sampling : after(15, sec)
    sampling -> normal : sampling_done
  state feeding_wasting_sampling [parallel]
    settings: executionOrder=1
    state feeding
      state inflow
        state inflow_act
          entry: act_pump_inflow(reac_ind)=p.max_pump_flow;
          vol_pump_in = floor(vol_pump_in/p.pump_res)*p.pump_res;
        state inflow_inact
          entry: act_pump_inflow=zeros(4,1);
          [vol_pump_in, reac_ind] = max(des_vol);
          during: [vol_pump_in, reac_ind] = max(des_vol);
        inflow_act -> inflow_inact [order 1] : after(vol_pump_in/p.max_pump_flow,sec)
        inflow_act -> inflow_inact [order 2] : [vol_pump_in<=0]
        inflow_inact -> inflow_act [order 2] : [vol_pump_in>=p.pump_res]
    state outflow_waste
      state outflow_act
        entry: act_pump_outflow(reac_ind)=...
        p.max_pump_flow;
        vol_pump_out = reactor_vol(reac_ind);
        % vol_pump_out = floor(reactor_vol(reac_ind)/...
        % p.pump_res)*p.pump_res;
      state outflow_inact
        entry: act_pump_outflow=zeros(4,1);
      feeding_wasting_sampling.outflow_waste.outflow_act -> feeding_wasting_sampling.outflow_waste.outflow_inact [order 1] : [vol_pump_out<=0]
      feeding_wasting_sampling.outflow_waste.outflow_act -> feeding_wasting_sampling.outflow_waste.outflow_inact [order 2] : after(vol_pump_out/p.max_pump_flow,sec)
      feeding_wasting_sampling.outflow_waste.outflow_inact -> feeding_wasting_sampling.outflow_waste.outflow_act [order 2] : {reac_ind = reac_ind+1;}
    state cleaning_procedure
    state outflow_sampling
      state outflow_act
        entry: vol_pump_out=p.pump_res;
        act_pump_outflow(reac_ind)=p.max_pump_flow;
      state outflow_inact
        entry: act_pump_outflow=zeros(4,1);
      feeding_wasting_sampling.outflow_sampling.outflow_act -> feeding_wasting_sampling.outflow_sampling.outflow_inact : after(vol_pump_out/p.max_pump_flow,sec)
      feeding_wasting_sampling.outflow_sampling.outflow_inact -> feeding_wasting_sampling.outflow_sampling.outflow_act [order 2] : {reac_ind=reac_ind+1;}
    (junction 263) -> inflow_inact [order 2] : [in(procedures.normal)]
    inflow_inact -> feeding_wasting_sampling.outflow_waste.outflow_act [order 1] : [sum(reactor_vol>p.waste_threshold)>0]{reac_ind=1;}
    cleaning_procedure -> (junction 263) : after(p.clean_time,sec)
    (junction 263) -> feeding_wasting_sampling.outflow_sampling.outflow_act [order 1] : [in(procedures.sampling)]{reac_ind=1;}
    feeding_wasting_sampling.outflow_sampling.outflow_inact -> cleaning_procedure [order 1] : [reac_ind==4]{send(sampling_done,procedures)}
    feeding_wasting_sampling.outflow_waste.outflow_inact -> cleaning_procedure [order 1] : [reac_ind == 4]
  (default) -> inflow_inact
  data: act_pump_inflow output =[0;0;0;0]; reactor_vol input; des_vol input size=4; vol_pump_in local; act_pump_outflow output =[0;0;0;0]; vol_pump_out local; sampling_req local; p parameter; reac_ind local =1
  events: sampling_done local FUNCTION_CALL_EVENT

== stateflow chart mdl_4reac/ 1 pump highest demand strategy feeding one rev only ==
  state procedures [parallel]
    settings: executionOrder=2
    state normal
    state sampling
      entry: sampling_req=true;
    (default) -> normal
    normal -> sampling : after(15, sec)
    sampling -> normal : sampling_done
  state feeding_wasting_sampling [parallel]
    settings: executionOrder=1
    state feeding
      state inflow
        state inflow_act
          entry: act_pump_inflow(reac_ind)=p.max_pump_flow;
        state inflow_inact
          entry: act_pump_inflow=zeros(4,1);
          [vol_pump_in, reac_ind] = max(des_vol);
          during: [vol_pump_in, reac_ind] = max(des_vol);
        inflow_act -> inflow_inact [order 1] : after(p.pump_res/p.max_pump_flow,sec)
        inflow_act -> inflow_inact [order 2] : [vol_pump_in<=0]
        inflow_inact -> inflow_act [order 2] : [vol_pump_in>=p.pump_res]
    state outflow_waste
      state outflow_act
        entry: act_pump_outflow(reac_ind)=...
        p.max_pump_flow;
        vol_pump_out = reactor_vol(reac_ind);
        % vol_pump_out = floor(reactor_vol(reac_ind)/...
        % p.pump_res)*p.pump_res;
      state outflow_inact
        entry: act_pump_outflow=zeros(4,1);
      feeding_wasting_sampling.outflow_waste.outflow_act -> feeding_wasting_sampling.outflow_waste.outflow_inact [order 1] : [vol_pump_out<=0]
      feeding_wasting_sampling.outflow_waste.outflow_act -> feeding_wasting_sampling.outflow_waste.outflow_inact [order 2] : after(vol_pump_out/p.max_pump_flow,sec)
      feeding_wasting_sampling.outflow_waste.outflow_inact -> feeding_wasting_sampling.outflow_waste.outflow_act [order 2] : {reac_ind = reac_ind+1;}
    state cleaning_procedure
    state outflow_sampling
      state outflow_act
        entry: vol_pump_out=p.pump_res;
        act_pump_outflow(reac_ind)=p.max_pump_flow;
      state outflow_inact
        entry: act_pump_outflow=zeros(4,1);
      feeding_wasting_sampling.outflow_sampling.outflow_act -> feeding_wasting_sampling.outflow_sampling.outflow_inact : after(vol_pump_out/p.max_pump_flow,sec)
      feeding_wasting_sampling.outflow_sampling.outflow_inact -> feeding_wasting_sampling.outflow_sampling.outflow_act [order 2] : {reac_ind=reac_ind+1;}
    (junction 263) -> inflow_inact [order 2] : [in(procedures.normal)]
    inflow_inact -> feeding_wasting_sampling.outflow_waste.outflow_act [order 1] : [sum(reactor_vol>p.waste_threshold)>0]{reac_ind=1;}
    cleaning_procedure -> (junction 263) : after(p.clean_time,sec)
    (junction 263) -> feeding_wasting_sampling.outflow_sampling.outflow_act [order 1] : [in(procedures.sampling)]{reac_ind=1;}
    feeding_wasting_sampling.outflow_sampling.outflow_inact -> cleaning_procedure [order 1] : [reac_ind==4]{send(sampling_done,procedures)}
    feeding_wasting_sampling.outflow_waste.outflow_inact -> cleaning_procedure [order 1] : [reac_ind == 4]
  (default) -> inflow_inact
  data: act_pump_inflow output =[0;0;0;0]; reactor_vol input; des_vol input size=4; vol_pump_in local; act_pump_outflow output =[0;0;0;0]; vol_pump_out local; sampling_req local; p parameter; reac_ind local =1
  events: sampling_done local FUNCTION_CALL_EVENT

== stateflow chart mdl_4reac/2 pumps highest demand strategy one rev ==
  state procedures [parallel]
    settings: executionOrder=1
    state normal
    state sampling
      entry: sampling_req=true;
    (default) -> normal
    normal -> sampling : after(15, sec)
    sampling -> normal : sampling_done
  state feeding [parallel]
    settings: executionOrder=2
    state inflow
      state inflow_act
        entry: act_pump_inflow(reac_ind_inflow)=...
        p.max_pump_flow;
      state inflow_inact
        entry: act_pump_inflow=zeros(4,1);
        [vol_pump_in, reac_ind_inflow] = max(des_vol);
        during: [vol_pump_in, reac_ind_inflow] = max(des_vol);
      inflow_act -> inflow_inact : after(p.pump_res/p.max_pump_flow,sec)
      inflow_inact -> inflow_act : [vol_pump_in>=p.pump_res]
    (default) -> inflow_inact
  state wasting_sampling [parallel]
    settings: executionOrder=3
    state outflow_waste
      state outflow_act
        entry: act_pump_outflow(reac_ind_outflow)=...
        p.max_pump_flow;
      state outflow_inact
        entry: act_pump_outflow=zeros(4,1);
        [vol_pump_out, reac_ind_outflow] = max(reactor_vol);
        during: [vol_pump_out, reac_ind_outflow] = ...
        max(reactor_vol);
      wasting_sampling.outflow_waste.outflow_act -> wasting_sampling.outflow_waste.outflow_inact [order 1] : after(vol_pump_out/p.max_pump_flow,sec)
      wasting_sampling.outflow_waste.outflow_act -> wasting_sampling.outflow_waste.outflow_inact [order 2] : [vol_pump_out<=0]
      wasting_sampling.outflow_waste.outflow_inact -> wasting_sampling.outflow_waste.outflow_act [order 2] : [vol_pump_out>=p.pump_res]
    state cleaning_procedure
    state outflow_sampling
      state outflow_act
        entry: vol_pump_out=p.pump_res;
        act_pump_outflow(reac_ind_outflow)=p.max_pump_flow;
      state outflow_inact
        entry: act_pump_outflow=zeros(4,1);
      wasting_sampling.outflow_sampling.outflow_act -> wasting_sampling.outflow_sampling.outflow_inact : after(vol_pump_out/p.max_pump_flow,sec)
      wasting_sampling.outflow_sampling.outflow_inact -> wasting_sampling.outflow_sampling.outflow_act [order 2] : {reac_ind_outflow=reac_ind_outflow+1;}
    (default) -> wasting_sampling.outflow_waste.outflow_inact
    wasting_sampling.outflow_waste.outflow_inact -> cleaning_procedure [order 1] : [in(procedures.sampling)]
    wasting_sampling.outflow_sampling.outflow_inact -> wasting_sampling.outflow_waste.outflow_inact [order 1] : [reac_ind_outflow==4]{send(sampling_done,procedures)}
    cleaning_procedure -> (junction 263) : after(p.clean_time,sec)
    (junction 263) -> wasting_sampling.outflow_sampling.outflow_act : {reac_ind_outflow=1;}
  data: act_pump_inflow output =[0;0;0;0]; reactor_vol input; des_vol input size=4; vol_pump_in local; act_pump_outflow output =[0;0;0;0]; vol_pump_out local; reac_ind_inflow local =1; sampling_req local; p parameter; reac_ind_outflow local =1
  events: sampling_done local FUNCTION_CALL_EVENT

== stateflow chart mdl_4reac/2 pumps highest demand strategy ==
  state procedures [parallel]
    settings: executionOrder=1
    state normal
    state sampling
      entry: sampling_req=true;
    (default) -> normal
    normal -> sampling : after(15, sec)
    sampling -> normal : sampling_done
  state feeding [parallel]
    settings: executionOrder=2
    state inflow
      state inflow_act
        entry: act_pump_inflow(reac_ind_inflow)=...
        p.max_pump_flow;
        vol_pump_in = floor(vol_pump_out/p.pump_res)...
        *p.pump_res;
      state inflow_inact
        entry: act_pump_inflow=zeros(4,1);
        [vol_pump_in, reac_ind_inflow] = max(des_vol);
        during: [vol_pump_in, reac_ind_inflow] = max(des_vol);
      inflow_act -> inflow_inact [order 1] : after(vol_pump_in/p.max_pump_flow,sec)
      inflow_act -> inflow_inact [order 2] : [vol_pump_in<=0]
      inflow_inact -> inflow_act : [vol_pump_in>=p.pump_res]
    (default) -> inflow_inact
  state wasting_sampling [parallel]
    settings: executionOrder=3
    state outflow_waste
      state outflow_act
        entry: act_pump_outflow(reac_ind_outflow)=...
        p.max_pump_flow;
        % vol_pump_out = floor(vol_pump_out/p.pump_res)...
        % *p.pump_res;
      state outflow_inact
        entry: act_pump_outflow=zeros(4,1);
        [vol_pump_out, reac_ind_outflow] = max(reactor_vol);
        during: [vol_pump_out, reac_ind_outflow] = ...
        max(reactor_vol);
      wasting_sampling.outflow_waste.outflow_act -> wasting_sampling.outflow_waste.outflow_inact [order 1] : after(vol_pump_out/p.max_pump_flow,sec)
      wasting_sampling.outflow_waste.outflow_act -> wasting_sampling.outflow_waste.outflow_inact [order 2] : [vol_pump_out<=0]
      wasting_sampling.outflow_waste.outflow_inact -> wasting_sampling.outflow_waste.outflow_act [order 2] : [vol_pump_out>=p.pump_res]
    state cleaning_procedure
    state outflow_sampling
      state outflow_act
        entry: vol_pump_out=p.pump_res;
        act_pump_outflow(reac_ind_outflow)=p.max_pump_flow;
      state outflow_inact
        entry: act_pump_outflow=zeros(4,1);
      wasting_sampling.outflow_sampling.outflow_act -> wasting_sampling.outflow_sampling.outflow_inact : after(vol_pump_out/p.max_pump_flow,sec)
      wasting_sampling.outflow_sampling.outflow_inact -> wasting_sampling.outflow_sampling.outflow_act [order 2] : {reac_ind_outflow=reac_ind_outflow+1;}
    (default) -> wasting_sampling.outflow_waste.outflow_inact
    wasting_sampling.outflow_waste.outflow_inact -> cleaning_procedure [order 1] : [in(procedures.sampling)]
    wasting_sampling.outflow_sampling.outflow_inact -> wasting_sampling.outflow_waste.outflow_inact [order 1] : [reac_ind_outflow==4]{send(sampling_done,procedures)}
    cleaning_procedure -> (junction 263) : after(p.clean_time,sec)
    (junction 263) -> wasting_sampling.outflow_sampling.outflow_act : {reac_ind_outflow=1;}
  data: act_pump_inflow output =[0;0;0;0]; reactor_vol input; des_vol input size=4; vol_pump_in local; act_pump_outflow output =[0;0;0;0]; vol_pump_out local; reac_ind_inflow local =1; sampling_req local; p parameter; reac_ind_outflow local =1
  events: sampling_done local FUNCTION_CALL_EVENT
